simulink model "fs9_sim_sdr_v0"  (R2022b)
settings: Solver=ode4  StartTime=0.0  StopTime=dm.duration  FixedStep=dm.dt  RelTol=1e-3
PreLoadFcn:
  | addpath('./Common');
  | addpath('./design_tuning');
  | addpath('./sim_config');
  | addpath('./sim_analysis');
  | addpath('./fsw_init');
  | addpath('./mdls');
  | rads2rpm    = 60/(2*pi);  %rad/s to rpm
  | deg2rad     = pi/180;
  | set_mdl_variant;
InitFcn:
  | %b5g_init_param_sdr_v1;
model workspace (MAT data in the model file):
  RWModelType = 0
undefined symbols (not defined in the file or in its folder): dm, Eclipse, fsw, MagSc, mdl, PVeci, Qi2b, RateSc, SunSc
libraries: simulink x3, vrlib x2, aerolibtransform2 x1
(part 2 of 2)

== stateflow chart fs9_sim_sdr_v0/Manager & Control/AOCS_FSW ==
  state AOCS_MGR
    tcur = elapsed(sec);
    exec_ttc;
    state NM
      state NM_MGR [parallel]
        en,du:
        sun_direction_proc;
        eclipse_proc;
        settings: executionOrder=1
        state OFF
        state SUP
          en,du:
          GUIDANCE.set_sun_dir(sun_dir);
          sup_trans_count;
        state GAP
          gap_trans_count;
        state MAN
        state FIP
        (default) -> AOCS_MGR.NM.NM_MGR.OFF
        AOCS_MGR.NM.NM_MGR.OFF -> AOCS_MGR.NM.NM_MGR.GAP [order 2] : [C2]{A5}
        AOCS_MGR.NM.NM_MGR.OFF -> AOCS_MGR.NM.NM_MGR.SUP [order 1] : [C1]{A4}
        AOCS_MGR.NM.NM_MGR.GAP -> AOCS_MGR.NM.NM_MGR.SUP [order 1] : [C1]{A4}
        AOCS_MGR.NM.NM_MGR.SUP -> AOCS_MGR.NM.NM_MGR.GAP [order 1] : [C2]{A5}
        AOCS_MGR.NM.NM_MGR.FIP -> AOCS_MGR.NM.NM_MGR.GAP [order 3] : GO_HOME[C2]{A5}
        AOCS_MGR.NM.NM_MGR.GAP -> AOCS_MGR.NM.NM_MGR.MAN [order 2] : SWITCH_MAN[C3]{A2}
        AOCS_MGR.NM.NM_MGR.SUP -> AOCS_MGR.NM.NM_MGR.MAN [order 2] : SWITCH_MAN[C3]{A2;}
        AOCS_MGR.NM.NM_MGR.FIP -> AOCS_MGR.NM.NM_MGR.SUP [order 2] : GO_HOME[C1]{A4}
        AOCS_MGR.NM.NM_MGR.FIP -> AOCS_MGR.NM.NM_MGR.MAN [order 1] : SWITCH_MAN[C3]{A2}
        AOCS_MGR.NM.NM_MGR.MAN -> AOCS_MGR.NM.NM_MGR.FIP : [C4]{A3}
      state GUIDANCE [parallel]
        settings: executionOrder=2
        state OFF
        state GAP
          en,du:
          gap_proc;
        state SUP
          en,du:
          gap_proc;
          %sup_proc;
        state MAN
          en,du:
          man_proc;
        state FIP
          fip_proc;
        (default) -> AOCS_MGR.NM.GUIDANCE.OFF
        AOCS_MGR.NM.GUIDANCE.OFF -> AOCS_MGR.NM.GUIDANCE.SUP [order 2] : SWITCH_SUP{A1}
        AOCS_MGR.NM.GUIDANCE.OFF -> AOCS_MGR.NM.GUIDANCE.GAP [order 1] : SWITCH_GAP{A2}
        AOCS_MGR.NM.GUIDANCE.GAP -> AOCS_MGR.NM.GUIDANCE.SUP [order 1] : SWITCH_SUP{A1}
        AOCS_MGR.NM.GUIDANCE.SUP -> AOCS_MGR.NM.GUIDANCE.GAP [order 1] : SWITCH_GAP{A2}
        AOCS_MGR.NM.GUIDANCE.FIP -> AOCS_MGR.NM.GUIDANCE.GAP [order 2] : SWITCH_GAP{A2}
        AOCS_MGR.NM.GUIDANCE.GAP -> AOCS_MGR.NM.GUIDANCE.MAN [order 2] : SWITCH_MAN{A3}
        AOCS_MGR.NM.GUIDANCE.FIP -> AOCS_MGR.NM.GUIDANCE.SUP [order 3] : SWITCH_SUP{A1}
        AOCS_MGR.NM.GUIDANCE.SUP -> AOCS_MGR.NM.GUIDANCE.MAN [order 2] : SWITCH_MAN{A3}
        AOCS_MGR.NM.GUIDANCE.FIP -> AOCS_MGR.NM.GUIDANCE.MAN [order 1] : SWITCH_MAN{A3}
        AOCS_MGR.NM.GUIDANCE.MAN -> AOCS_MGR.NM.GUIDANCE.FIP : SWITCH_FIP{A4}
      state NM_CONTROL [parallel]
        settings: executionOrder=3
        state WHEEL_ONLY
          en, du:
          pre_proc;
          wheel_control_proc;
          wheel_off_loading_proc;
        state OFF
        (default) -> AOCS_MGR.NM.NM_CONTROL.OFF
        AOCS_MGR.NM.NM_CONTROL.OFF -> WHEEL_ONLY
    state ASH_MGR
      state ASH [parallel]
        du:
        ASH_MGR_RTC;
        settings: executionOrder=1
        state IDLE
        state STABILIZE
          entry, during:
          stabilize_processing;
        state SLO
          entry,during:
          sun_lock_processing;
          wheel_off_loading_proc
          if ~sun_presence
          count_day_night =  count_day_night+1;
          else
          count_day_night = 0;
          end
        state STRA
          during:
          if sun_presence
          count_day_night =  count_day_night+1;
          else
          count_day_night = 0;
          end
        (default) -> IDLE
        IDLE -> STABILIZE : [C1]{A1}
        STABILIZE -> STRA : [C2]{A2}
        STRA -> SLO : [C3]{A3}
        SLO -> STRA : [C4]{A4}
      state ASH_CTRL [parallel]
        du:
        ASH_CTRL_RTC
        settings: executionOrder=2
        state OFF
        state MTQ_ONLY
          entry, during:
          RW_FUN   = ...
          rw_momentum_control(SENSOR_IN.Hrw);
          MTQ_FUN = ...
          magnetic_control(SENSOR_IN.MAG_FUNC)
          exit:
          MTQ_FUN = zeros(3,1);
        state MTQ_AND_RW
          entry,during:
          RW_FUN = ...
          sunsensor_control(SENSOR_IN.SS_FUNC,...
          SENSOR_IN.rate_est );
        (default) -> AOCS_MGR.ASH_MGR.ASH_CTRL.OFF
        AOCS_MGR.ASH_MGR.ASH_CTRL.OFF -> MTQ_ONLY : SCHEDULE_OBJECT
        MTQ_ONLY -> MTQ_AND_RW : SELECT_MTQ_AND_RW
        MTQ_AND_RW -> MTQ_ONLY : SELECT_MTQ_ONLY
      state rw_cmd = rw_momentum_control(HrwEst) [function]
      state stop_sim [function]
      state mtq_cmd = magnetic_control(MAG_FUNC) [function]
      state rw_cmd = sunsensor_control(ss_tm,iru_tm) [function]
    (default) -> (junction 132)
    (junction 132) -> (junction 135) [order 2]
    (junction 132) -> NM [order 1] : [AOCS_MODE==1]
    (junction 135) -> ASH_MGR
  data: C function_output; C function_output; C function_output; C function_output; sat_in_eclipse local boolean size=1 =false; object_state local Enum: NMMODE size=1 =NMMODE.OFF; sun_dir local double size=3 =[1 0 0]'; gap_sup_counter local double size=1 =0; steady_count local double size=1 =0; sup_gap_counter local double size=1 =0; dt function_output; C function_output; C function_output; Q function_output; W function_output; A function_output; sv function_input; qin function_input; dt function_input; object_state local Enum: GUIDMODE size=1 =GUIDMODE.OFF; sun_dir local double size=3 =[1 0 0]';; Qin2cons local double size=4 =[1 0 0 0]';; Wcons local double size=3 =[0 0 0]'; Acons local double size=3 =[0 0 0]'; Qlvlh2cons_end local double size=4 =[1 0 0 0]'; dt_man local double size=1 =0; man_feasibility_flag local boolean size=1 =false; theta_rot local double size=1 =0; Amax local double size=1 =0; end_of_man_flag local boolean size=1 =false; t_curr local double size=1 =0; Acurr local double size=1 =0; Wcurr local double size=1 =0; theta_curr local size=1 =0; Qlvlh2cons_fip local double size=4 =[1 0 0 0]'; Qin2sat_init local double size=4 =[1 0 0 0]'; T_VHF local double size=1 =fsw.dt; axis_rot local double size=3 =[1 0 0]'; T1 local double size=1 =0; T2 local double size=1 =0; Wrot local double size=1 =0; da function_output; dr function_output; Hrw local double size=3 =[0 0 0]'; Qerr local double size=4 =[1 0 0 0]'; d_theta local double size=3 =[0 0 0]'; d_omega local double size=3 =[0 0 0]'; Acons local double size=3 =[0 0 0]'; Wcons local double size=3 =[0 0 0]'; Qin2cons local double size=4 =[1 0 0 0]'; West local double size=3 =[0 0 0]'; rate_bias local double size=3 =[0 0 0]'; B0 local double size=3 =[0 0 0]'; maxB local double size=1; C function_output boolean size=1; HrwEst function_input double size=3; rw_cmd function_output; C function_output; MAG_FUNC function_input double size=9; mtq_cmd function_output; C function_output; ss_tm function_input double size=4; iru_tm function_input double size=3; rw_cmd function_output; C function_output; object_state local Enum: ASHMODE size=1; tcur local double size=1 =0; fsw parameter; count_stab local double size=1; count_day_night local double size=1 =0; SENSOR_IN input Bus: SENSORS; stabilized local boolean size=1; stabilize_duration local double; sun_mislocked_duration local double size=1 =0; sun_locked_duration local double size=1 =0; sun_presence local boolean size=1 =false; RW_FUN output double size=3 =zeros(3,1); MTQ_FUN output double size=3 =zeros(3,1); AOCS_MODE local double size=1 =fsw.aocs_mode; udot_norm local double size=1 =0
  data udot_norm settings: description=log data
  events: SWITCH_MAN local FUNCTION_CALL_EVENT; GO_HOME local FUNCTION_CALL_EVENT; SWITCH_SUP local FUNCTION_CALL_EVENT; SWITCH_GAP local FUNCTION_CALL_EVENT; SWITCH_MAN local FUNCTION_CALL_EVENT; SWITCH_FIP local FUNCTION_CALL_EVENT; SELECT_MTQ_AND_RW local FUNCTION_CALL_EVENT; SELECT_MTQ_ONLY local FUNCTION_CALL_EVENT; SCHEDULE_OBJECT local FUNCTION_CALL_EVENT
  function C = C1:
    | function C = C1
    | C = sat_in_eclipse== false;
  function C = C2:
    | function C = C2
    | C = sat_in_eclipse== true;
  function C = C3:
    | function C = C3
    | C = GUIDANCE.get_man_feasibility_flag;
  function C = C4:
    | function C = C4
    | C = GUIDANCE.get_end_of_man_flag;
  function A2:
    | function A2
    | send(GUIDANCE.SWITCH_MAN, GUIDANCE);
    | object_state = NMMODE.MAN;
  function A3:
    | function A3
    | 
    | send(GUIDANCE.SWITCH_FIP, GUIDANCE);
    | object_state = NMMODE.FIP;
  function A4:
    | function A4
    | send(GUIDANCE.SWITCH_SUP, GUIDANCE);
    | object_state = NMMODE.SUP;
    | sup_gap_counter = 0;
  function A5:
    | function A5
    | 
    | send(GUIDANCE.SWITCH_GAP, GUIDANCE);
    | object_state = NMMODE.GAP;
    | gap_sup_counter = 0;
  function eclipse_proc:
    | function eclipse_proc
    | 
    | p_sat_eci = SENSOR_IN.pvt_eci_nav(1:3);
    | 
    | if dot(p_sat_eci, sun_dir) > fsw.nm_mgr.eclipse_param
    |     sat_in_eclipse = false;
    | else
    |     sat_in_eclipse = true;
    | end
  function sun_direction_proc:
    | function sun_direction_proc
    | jD = SENSOR_IN.pvt_eci_nav(7);
    | T = JDCentury(jD);
    | lamda_mean     = rem(280.460+36000.771*T,360);
    | mean_anomaly   = rem(357.5291092+35999.05034*T,360);
    | lamda_ecliptic = lamda_mean+ 1.914666471*sind(mean_anomaly)...
    |                  + 0.019994643*sind(2*mean_anomaly);
    | % Obliquity of ecliptic
    | epsilon = 23.439291 -0.0130042*T;
    | sun_dir  = [cosd(lamda_ecliptic);...
    |            cosd(epsilon)*sind(lamda_ecliptic);...
    |            sind(epsilon)*sind(lamda_ecliptic)];
  function sup_trans_count:
    | function sup_trans_count
    | [ang_err, ~] = NM_CONTROL.get_control_error;
    | ang_max = max(abs(ang_err));
    | if ang_max >= fsw.nm_mgr.ang_thd
    |     gap_sup_counter = gap_sup_counter + fsw.dt;
    |     if steady_count ~= 0
    |         steady_count = 0;
    |     end
    | else
    |      if steady_count <=  fsw.nm_mgr.Tsteady
    |          gap_sup_counter = gap_sup_counter + fsw.dt;
    |          steady_count    = steady_count + fsw.dt;
    |      else
    |          gap_sup_counter = 0;
    |      end
    | end
  function gap_trans_count:
    | function gap_trans_count
    | [ang_err, ~] = NM_CONTROL.get_control_error;
    | ang_max = max(abs(ang_err));
    | if ang_max >= fsw.nm_mgr.ang_thd
    |     sup_gap_counter = sup_gap_counter + fsw.dt;
    |     if steady_count ~= 0
    |         steady_count = 0;
    |     end
    | else
    |      if steady_count <=  fsw.nm_mgr.Tsteady
    |          sup_gap_counter = sup_gap_counter + fsw.dt;
    |          steady_count    = steady_count + fsw.dt;
    |      else
    |          sup_gap_counter = 0;
    |      end
    | end
  function dt = make_fesability:
    | function dt = make_fesability
    |  
    | Qi2bInit   = SENSOR_IN.qi2b_est;
    | Qi2l       = SENSOR_IN.nav_out(4:7);
    | Isat       = fsw.EstIb;
    | G          = fsw.rw.func.G;
    | DHalloc    = fsw.guid.WHEEL_MOM_ALLOC;
    | TrwMax     = fsw.guid.WHEEL_MAX_TORQUE;
    | Wthd       = fsw.guid.MAN_ANG_RATE_SAT;
    | 
    | Qi2consEnd = QMul(Qi2l, Qlvlh2cons_end);
    | 
    | Qman       = QMul(QInv(Qi2bInit), Qi2consEnd);
    | Qman       = QNormal(Qman);
    | 
    | if Qman(1) <0
    |     Qman = -Qman;
    | end
    | theta_rot = 2 * acos(Qman(1));
    | 
    | if theta_rot < fsw.guid.EPSILON_MAN
    |     theta_rot = 0;
    |     axis_rot  =[1 0 0]';
    | else
    |     axis_rot = Qman(2:4)/sqrt(1-Qman(1)^2);
    | end
    | 
    | Acc         = abs(G*Isat*axis_rot);
    | dh_over_a   = [inf inf inf inf]';
    | tmax_over_a = [inf inf inf inf]';
    | for i=1:4
    |     if Acc(i)~=0
    |         dh_over_a(i)  = DHalloc(i)/Acc(i);
    |         tmax_over_a(i)= TrwMax(i)/Acc(i);
    |     end
    | end
    | Wmax = min([dh_over_a' Wthd]);
    | Amax = min(tmax_over_a);
    | 
    | %% step 4 
    | if theta_rot <= Wmax^2/Amax
    |     dt = sqrt(4*theta_rot/Amax);
    | else
    |     dt = (theta_rot/Wmax+Wmax/Amax); %(theta_rot+Wmax^2/Amax)/Wmax
    | end
    | dt    = ceil(dt);
    | 
    | end
  function C = get_end_of_man_flag:
    | function C = get_end_of_man_flag
    |  
    | C = end_of_man_flag;
  function C = get_man_feasibility_flag:
    | function C = get_man_feasibility_flag
    | if dt_man == 0
    |    fprintf('dt_man: ');
    |    dt_man  = make_fesability;
    |    fprintf('%.1f, ',dt_man);
    |    check_man_feasibility_proc;
    |    while (~man_feasibility_flag)
    |        dt_man = dt_man+1;
    |        check_man_feasibility_proc;
    |        fprintf('%.1f, ',dt_man);
    |    end
    |    fprintf('\n');
    | end
    | check_man_feasibility_proc;
    | C = man_feasibility_flag;
  function [Q, W, A] = get_guid_data:
    | function [Q, W, A]=get_guid_data
    | A = Acons;    
    | Q = Qin2cons ;
    | W = Wcons ;   
    | end
  function set_sun_dir(sv):
    | function set_sun_dir(sv)
    | sun_dir = sv;
  function set_man_profile(qin, dt):
    | function set_man_profile(qin, dt)
    | Qlvlh2cons_end    = qin;
    | dt_man            = dt;
    | end
  function check_man_feasibility_proc:
    | function check_man_feasibility_proc
    | 
    | Isat    = fsw.EstIb;
    | G       = fsw.rw.func.G;
    | DHalloc = fsw.guid.WHEEL_MOM_ALLOC;
    | TrwMax  = fsw.guid.WHEEL_MAX_TORQUE;
    | Wthd    = fsw.guid.MAN_ANG_RATE_SAT;
    | Omega   = SENSOR_IN.nav_out(1:3);
    | 
    | Qlvlh_init2end = [cos(Omega(2)*dt_man/2); 0;...
    |                   sin(Omega(2)*dt_man/2); 0];
    | 
    | Qin2lvlh       = SENSOR_IN.nav_out(4:7);
    | 
    | Qin2cons_end   = QMul(QMul(Qin2lvlh, Qlvlh_init2end), Qlvlh2cons_end);
    | Qin2sat_init   = SENSOR_IN.qi2b_est;
    | Qman           = QMul(QInv(Qin2sat_init), Qin2cons_end);
    | Qman           = QNormal(Qman);
    | 
    | if Qman(1) <0
    |         Qman = -Qman;
    | end
    | 
    | if Qman(1) > 1 
    |     man_feasibility_flag = false;
    |     return;
    | end
    | 
    | theta_rot = 2 * acos(Qman(1));
    | 
    | if theta_rot < fsw.guid.EPSILON_MAN
    |     theta_rot = 0;
    |     axis_rot  =[1 0 0]';
    | else
    |     axis_rot = Qman(2:4)/sqrt(1-Qman(1)^2);
    | end
    | 
    | Acc         = abs(G*Isat*axis_rot);
    | dh_over_a   = [inf inf inf inf]';
    | tmax_over_a = [inf inf inf inf]';
    | for i=1:4
    |     if Acc(i)~=0
    |         dh_over_a(i)  = DHalloc(i)/Acc(i);
    |         tmax_over_a(i)= TrwMax(i)/Acc(i);
    |     end
    | end
    | Wmax = min([dh_over_a' Wthd]);
    | Amax = min(tmax_over_a);
    | 
    | if dt_man < fsw.dt || Amax == 0
    |     man_feasibility_flag = false;
    |     
    | elseif dt_man <= 2*Wmax/Amax && theta_rot<=Amax*dt_man^2/4
    |     man_feasibility_flag = true;
    |     
    | elseif dt_man >= 2*Wmax/Amax && theta_rot<=Wmax*dt_man-Wmax^2/Amax
    |     man_feasibility_flag = true;
    |     
    | else
    |     man_feasibility_flag = false;
    | end
    | 
    | % if(~man_feasibility_flag)
    | %     disp('MAN Failed');
    | % end
  function man_proc:
    | function man_proc
    | 
    | if t_curr >= dt_man
    |     Acurr = 0;
    |     Wcurr = 0;
    |     theta_curr = theta_rot;
    |     end_of_man_flag = true;
    | elseif t_curr >= T2 && t_curr < dt_man
    |     Acurr = -Amax;
    |     Wcurr = Amax*(dt_man - t_curr);
    |     theta_curr = theta_rot - 0.5*Amax * (dt_man - t_curr)^2;
    |  elseif t_curr >= T1 && t_curr < T2
    |     Acurr = 0;
    |     Wcurr = Wrot;
    |     theta_curr = theta_rot/2 + Wrot * (t_curr - dt_man/2);
    | elseif t_curr < T1
    |     Acurr = Amax;
    |     Wcurr = Amax * t_curr;
    |     theta_curr = 0.5*Amax * t_curr^2;
    | end    
    | Qsat2cons_curr = [cos(theta_curr/2);sin(theta_curr/2).*axis_rot];
    | Qin2cons = QMul(Qin2sat_init,Qsat2cons_curr);
    | Wcons = Wcurr.*axis_rot;
    | Acons = Acurr.*axis_rot;
    | t_curr = t_curr + T_VHF;
    |     
    | end
  function fip_proc:
    | function fip_proc
    | 
    | Qin2lvlh = SENSOR_IN.nav_out(4:7);
    | Qin2cons = QMul(Qin2lvlh, Qlvlh2cons_fip);
    | 
    | Worb = SENSOR_IN.nav_out(1:3);
    | 
    | q_temp = QMul(QMul(QInv(Qlvlh2cons_fip),[0;Worb]), Qlvlh2cons_fip);
    | Wcons  = q_temp(2:4);
    |     
    | end
  function gap_proc:
    | function gap_proc
    | Acons    = zeros(3,1);
    | Qin2cons = SENSOR_IN.nav_out(4:7);
    | Wcons    = SENSOR_IN.nav_out(1:3);
    | end
  function sup_proc:
    | function sup_proc()
    | 
    | if fsw.guid.SUP_SLEW_MODE
    |     Qin2cons = sun_sync_sup_slew;
    | else
    |     Qin2cons = dir_sup_slew;
    | end
    | Wcons = zeros(3,1);
    | Acons = zeros(3,1);
    | end
    | 
    | function QuatSup = sun_sync_sup_slew
    |     Qi2l = SENSOR_IN.nav_out(4:7);
    |     SunEci = sun_dir;
    |     Qorb = QMul(Qi2l,QMul([0 0 1 0]',QInv(Qi2l)));
    |     Norb = Qorb(2:4);
    |     Ux   = cross(Norb,SunEci);
    |     Ux   = Ux/norm(Ux);
    |     if(Ux(3)>0)
    |         Ux = -Ux;
    |     end
    |     Uz   = -SunEci;
    |     Uy   = cross(Uz,Ux);
    |     QuatSup = M2Q([Ux Uy Uz]);
    | end
    | 
    | 
    | function QuatSup = dir_sup_slew
    |     Qin2sat = SENSOR_IN.qi2b_est;
    |     SunEci  = sun_dir;
    |     Qsb = QMul(QInv(Qin2sat),QMul([0;SunEci],Qin2sat));
    |     SunBody = Qsb(2:4);
    |     prj = dot([0 0 -1]', SunBody);
    |     if prj >1 || prj< -1
    |         prj = 1;
    |     end
    |     dlt_ang = acos(prj);
    |     rotAxis = cross([0 0 -1]', SunBody);
    |     rotAxis = rotAxis/norm(rotAxis);
    |     Qb2c = [cos(dlt_ang/2); rotAxis*sin(dlt_ang/2)];
    |     QuatSup = QMul(Qin2sat,Qb2c);
    | end
  function A1:
    | function A1
    | 
    | object_state = GUIDMODE.SUP;
  function A2:
    | function A2
    | 
    | object_state = GUIDMODE.SUP;
  function A3:
    | function A3
    | 
    | object_state = GUIDMODE.MAN;
    | 
    | %% initialization of man proc
    | alpha  = 1 - sqrt(1 - 4*theta_rot/(Amax*dt_man^2));
    | T1     = alpha*dt_man/2;
    | T2     = dt_man-T1;
    | Wrot   = alpha * Amax *dt_man/2;
    | T1     = alpha*dt_man/2;
    | T2     = dt_man-T1;
    | Wrot   = alpha * Amax *dt_man/2;
    | end_of_man_flag = false;
    | t_curr = 0;
    | Qlvlh2cons_fip = Qlvlh2cons_end;
  function A4:
    | function A4
    | 
    | object_state = GUIDMODE.FIP;
    | Acons = zeros(3,1);
  function pre_proc:
    | function pre_proc()
    | Qin2sat = SENSOR_IN.qi2b_est;
    | West    = SENSOR_IN.rate_est;
    | Hrw     = SENSOR_IN.Hrw;
    | 
    | [Qin2cons, Wcons, Acons] = GUIDANCE.get_guid_data;
    | deltaQ = QMul(QInv(Qin2cons),Qin2sat);
    | if deltaQ(1)<0
    |         deltaQ = deltaQ *-1;
    | end
    | 
    | d_theta = 2.0*deltaQ(2:4);
    | d_omega = West-Wcons;
    | Qerr = QNormal(deltaQ);
    | 
    | end
  function wheel_off_loading_proc:
    | function wheel_off_loading_proc
    | Isat = fsw.EstIb;
    | B = SENSOR_IN.MAG_FUNC(7:9);
    | Htot = Isat*West + Hrw;
    | % delta_h = (Hrw + fsw.Ib*RateEst) - fsw.rw.func.h_ref;
    | delta_h = Htot - fsw.ctrl.h_ref;
    | m = cross(B,delta_h)*(-fsw.ctrl.off_load_ctrl_gain/norm(B)^2);
    | m_max = max(abs(m));
    | if m_max  > fsw.mtq.func.max_dipole
    |     m = m*(fsw.mtq.func.max_dipole/m_max) ;
    | end
    |     
    | MTQ_FUN = m;
    | end
  function wheel_control_proc:
    | function wheel_control_proc
    | Kv = fsw.ctrl.KD;
    | Ke = fsw.ctrl.KP;
    | Isat = fsw.EstIb;
    | % if Qerr(1)==1
    | %     disp('divided by zeros');
    | % end
    | if dot(Qerr(2:4),Qerr(2:4)) > 0.25 * fsw.ctrl.thet_thd^2
    |    if Qerr(1)==1
    |        B0 = zeros(3,1);
    |    else
    |        Bdir = Qerr(2:4)/norm(Qerr(2:4));
    |        B0 = -fsw.ctrl.RateBiasMaxNorm*Bdir;
    | %        B0 = -(fsw.ctrl.RateBiasMaxNorm/sqrt(1-Qerr(1)^2)).*Qerr(2:4);
    | %        disp(Qerr(2:4));
    |    end
    |    maxB = max([1;abs(B0)./fsw.ctrl.RateBiasMax]);
    |    rate_bias = B0/maxB;  
    |    Trw = Isat*(Kv.*(d_omega - rate_bias));
    |    Tol = zeros(3,1);
    | else
    |    rate_bias = zeros(3,1);
    |    Trw = Isat*(Ke.*d_theta + Kv.*d_omega); 
    |    Tol  = Isat*Acons + cross(Wcons, Isat*Wcons + Hrw);
    | end
    | 
    | RW_FUN = Trw - Tol;
    | 
    | end
  function [da ,dr] = get_control_error:
    | function [da ,dr] = get_control_error
    | da = d_theta;
    | dr = d_omega;
  function stabilize_processing:
    | function stabilize_processing
    | 
    | udot = SENSOR_IN.MAG_FUNC(1:3);
    | udot_norm = norm(udot);
    | 
    | if  udot_norm < fsw.ash_mgr.epsilon
    |     count_stab = count_stab+1;
    | else
    |     count_stab = 0;
    | end
    | if count_stab > fsw.ash_mgr.Tstab
    |     stabilized = true;
    |     if fsw.ash_mgr.stop_once_stab
    |         stop_sim;
    |     end
    | end
  function A1:
    | function A1
    | 
    | count_stab = 0;
    | stabilized = false;
    | stabilize_duration = 0;
    | send(ASH_CTRL.SCHEDULE_OBJECT, ASH_CTRL.OFF);
    | 
    | 
    | ASH_MGR.object_state = ASHMODE.STAB;
  function C = C1:
    | function C = C1
    | % Check that all necessary equipments for the STABILIZE submode are ON
    | C = true;
  function ASH_CTRL_RTC:
    | function ASH_CTRL_RTC
    | 
    | if ~in(ASH_CTRL.MTQ_AND_RW)
    |     sunsensor_control(SENSOR_IN.SS_FUNC, SENSOR_IN.rate_est );
    | end
  function sun_lock_processing:
    | function sun_lock_processing
    | 
    | sun_locked_duration = sun_locked_duration + 1;
  function C = C2:
    | function C = C2
    | C = stabilized;%stablized;
  function A2:
    | function A2
    | ASH_MGR.object_state = ASHMODE.STRA;
    | count_day_night = 0;
  function wheel_off_loading_proc:
    | function wheel_off_loading_proc
    | 
    | West    = SENSOR_IN.rate_est;
    | Hrw     = SENSOR_IN.Hrw;
    | Isat = fsw.EstIb;
    | B = SENSOR_IN.MAG_FUNC(7:9);
    | Htot = Isat*West + Hrw;
    | % delta_h = (Hrw + fsw.Ib*RateEst) - fsw.rw.func.h_ref;
    | delta_h = Htot - fsw.rw.func.h_ref;
    | m = cross(B,delta_h)*(-fsw.rw.func.off_load_ctrl_gain/norm(B)^2);
    | 
    | 
    | m_max = max(abs(m));
    | if m_max  > fsw.mtq.func.max_dipole
    |     m = m*(fsw.mtq.func.max_dipole/m_max) ;
    | end
    |         
    | MTQ_FUN = m/5;%@@
    | end
  function ASH_MGR_RTC:
    | function ASH_MGR_RTC
    | 
    | sun_presence = ...
    |     boolean(SENSOR_IN.SS_FUNC(4));
    | ASH_MGR.object_state = ...
    |     ASH_MGR.object_state;
    | 
    | % count_stab = count_stab;
  function C = C3:
    | function C = C3
    | C = count_day_night >= fsw.ash_mgr.Tconf;
  function A3:
    | function A3
    | 
    | % send(ASH_CTRL.SELECT_MTQ_AND_RW, ASH_CTRL.MTQ_ONLY);
    | ASH_MGR.object_state = ASHMODE.SLO;
    | count_day_night = 0;
    | 
    | sun_locked_duration = 0;
    | sun_mislocked_duration = 0;
  function C = C4:
    | function C = C4
    | C = count_day_night >= fsw.ash_mgr.Tconf;
  function A4:
    | function A4
    | 
    | % send(ASH_CTRL.SELECT_MTQ_ONLY, ASH_CTRL.MTQ_AND_RW);
    | % send(ASH_CTRL.SELECT_MTQ_AND_RW, ASH_CTRL.MTQ_ONLY);
    | % 
    | % send(ASH_CTRL.SELECT_MTQ_ONLY, ASH_CTRL.MTQ_AND_RW);
    | ASH_MGR.object_state = ASHMODE.STRA;
    | count_day_night = 0;
    | count_stab = 0;
    | stabilized = false;
  function exec_ttc:
    | function exec_ttc
    | if isempty(fsw.ttc)
    |     return;
    | end
    | ttc = fsw.ttc;
    | num = size(ttc,2);
    | % disp(elapsed('sec'));
    | for i=1:num
    |     if (ttc(i).exec_time == tcur)
    |         switch ttc(i).type
    |             case TTC.GO_HOME
    |                 fprintf('%.2f : GO HOME\n',tcur);
    |                 send(NM.NM_MGR.GO_HOME, NM.NM_MGR);
    |             case TTC.SWITCH_MAN
    |                 NM.GUIDANCE.set_man_profile(ttc(i).q_lvlh2cons, ttc(i).dt);
    |                 ra = asind(ttc(i).q_lvlh2cons(2:4))*2;
    |                 fprintf('%.2f : MAN (%.1f, %.1f, %.1f) in %.1f sec\n',...
    |                        tcur,ra(1), ra(2), ra(3), ttc(i).dt );
    |                 send(NM.NM_MGR.SWITCH_MAN, NM.NM_MGR);
    |         end
    |     end
    |  
    | end

== matlab function fs9_sim_sdr_v0/Space Environment Models/Eclipse Condition ==
  data: SunEci input; EclipFlag output; PvEci input
function EclipFlag  = Eclipse(SunEci, PvEci)
Dp = -PvEci(1:3)*1e-3;  % earth vector in Km
Rp = 6378.137;          % earth radius in km
Rs = 6.9599e5;          % solar photosphere radius in km
S  = 1.49597870e8;      % astronomical unit in km
C  = 1.385e6;           % size of earth shadow cone
Ds = (S.*SunEci + Dp);  % vector from S/C to the Sun

DsNorm = norm(Ds);
DpNorm = norm(Dp);
rho_s  = asind(Rs/DsNorm);
rho_p  = asind(Rp/DpNorm);
theta  = acosd(dot(Ds, Dp) / (DsNorm * DpNorm));
if ( theta < (rho_p - rho_s) && DsNorm > S && (S + C) > DsNorm)
    EclipFlag = 1;
else
	EclipFlag = 0;
end

== matlab function fs9_sim_sdr_v0/Space Environment Models/Sun Model ==
  data: jD input; SunEci output
function SunEci = SunModel(jD)
T = JDCentury(jD);
lamda_mean     = rem(280.460+36000.771*T,360);
mean_anomaly   = rem(357.5291092+35999.05034*T,360);
lamda_ecliptic = lamda_mean+ 1.914666471*sind(mean_anomaly)...
                 + 0.019994643*sind(2*mean_anomaly);
% Obliquity of ecliptic
epsilon = 23.439291 -0.0130042*T;
SunEci  = [cosd(lamda_ecliptic);...
           cosd(epsilon)*sind(lamda_ecliptic);...
           sind(epsilon)*sind(lamda_ecliptic)];

== matlab function fs9_sim_sdr_v0/Manager & Control/AOCS_FSW/AOCS_MGR.ASH_MGR.magnetic_control/Bdot Control ==
  settings: updateMethod=DISCRETE
  data: MAG_FUNC input; Mc output; fsw parameter
%% Bdot Control Rev
function Mc  = Bdot(MAG_FUNC, fsw)

sdot  =  MAG_FUNC(4:6);
Mc    = -fsw.bdot_gain.*sdot;

end

== matlab function fs9_sim_sdr_v0/NAV & IAE/NAVIGATION ==
  data: pvt_eci input; nav_out output; pvt_eci_nav output; fsw parameter
function [nav_out, pvt_eci_nav]  = Navgation(pvt_eci, fsw)

p_nav = pvt_eci(1:3) + fsw.nav.p_noise*randn(3,1)*fsw.nav.noise_enable;
v_nav = pvt_eci(4:6) + fsw.nav.v_noise*randn(3,1)*fsw.nav.noise_enable;

omega_orbit = OrbitPusaltion(pvt_eci);
Qi2l        = PVi2Qi2l(pvt_eci);
nav_out     = [omega_orbit; Qi2l];
pvt_eci_nav  = [p_nav ;v_nav;pvt_eci(7)];

== matlab function fs9_sim_sdr_v0/Manager & Control/AOCS_FSW/AOCS_MGR.ASH_MGR.sunsensor_control/SunAngErr ==
  data: deltaAngle_c2b output; snr_fun input
function deltaAngle_c2b = RPLD_CTRL_PROC(snr_fun)

if ~snr_fun(4) 
    deltaAngle_c2b = [0;0;0];
    return;
end

vec_sun_b = snr_fun(1:3);
mag = norm(vec_sun_b);
if mag~=0
    vec_sun_b = vec_sun_b/mag;
end

%% DCM to Euler Angle Method
zb = (-1)*vec_sun_b';
yb = [0 vec_sun_b(3) -vec_sun_b(2)];
xb = cross(yb,zb);
R_B2C = [xb;yb;zb];

theta_c2b = -asin(R_B2C(3, 1));
phi_c2b = atan(R_B2C(3, 2) / R_B2C(3, 3));
% psi_c2b = atan2(R_B2C(2, 1), R_B2C(1, 1)); //3.14
psi_c2b = atan(R_B2C(2, 1) / R_B2C(1, 1));

%% deltaAngle_c2b = deltaAngle_b/c = -deltaAngle_c/b = -deltaAngle_b2c
deltaAngle_c2b = [phi_c2b; theta_c2b; psi_c2b];

== matlab function fs9_sim_sdr_v0/NAV & IAE/Inertial Attitude Estimation ==
  settings: updateMethod=DISCRETE
  data: Qi2b_true input; Q2ib output; RateSc_true input; RateSc output; fsw parameter
function [Q2ib, RateSc]= IAE(Qi2b_true, RateSc_true, fsw)

if fsw.iae.noise_enable
    dltQ   = (fsw.iae.att_noise.*randn(3,1)/2)*fsw.iae.noise_enable;
    qNoise = [sqrt(1-dltQ'*dltQ);dltQ];
    Q2ib   = QUnit(QMul(Qi2b_true, qNoise));
else
    Q2ib   = Qi2b_true;
end
RateSc = RateSc_true + fsw.iae.rate_noise*randn(3,1)*fsw.iae.noise_enable;

== matlab function fs9_sim_sdr_v0/MTQ_FUN/MATLAB Function ==
  data: Mc input; duty output double; fsw parameter
function duty = fcn(Mc, fsw)
max_dipole = fsw.mtq.func.max_dipole;
mtq_period = fsw.mtq.cycle;
Mm = Mc;
mx = max(abs(Mc));
if mx>max_dipole
    Mm = Mm*(max_dipole/mx);
end

duty = Mm*(mtq_period-1)/(max_dipole*mtq_period);

== matlab function fs9_sim_sdr_v0/Sensor Modeling/ZARM FGM-A-75 ==
  settings: updateMethod=DISCRETE
  data: MagScTrue input; MagScNoise output; dm parameter
function MagScNoise = fcn(MagScTrue, dm)

if dm.mag_mdl.enable_noise

    mag_norm_ture = norm(MagScTrue);
    if abs(mag_norm_ture-eps) < 10*eps
        MagScNoise = MagScTrue;
        return;
    end
    mag_dir_true  = MagScTrue/mag_norm_ture;
    
    
    
    rdn_dir = [randn(2,1);0];        % only for x and y axis
    rdn_dir = rdn_dir/norm(rdn_dir);
    thet_dist = dm.mag_mdl.ang_err*randn(1,1)/2; %half noise
    
    q_dist = [cos(thet_dist); rdn_dir*sin(thet_dist)];
    
    mag_dir_dist = QMul([0;mag_dir_true],q_dist);
    mag_norm_dist = mag_norm_ture*(1 + dm.mag_mdl.norm_err*randn(1,1));
    
    mag_dist = mag_dir_dist(2:4)*mag_norm_dist;
    
    MagScNoise = mag_dist + dm.mag_mdl.noise * randn(3,1)...
                          + dm.mag_mdl.linerity_err * randn(3,1)...
                          + dm.mag_mdl.offset_err * randn(3,1);

else
    MagScNoise = MagScTrue;
end

== matlab function fs9_sim_sdr_v0/Spacecraft/Spacecraft Dynamics/Disturbance Models/Subsystem/Peci to Body ==
  data: Va input; Qa2b input; Vb output
function Vb = EciToBody(Va,Qa2b)
Qb2a = QInv(Qa2b);
qout = QMul(QMul(Qb2a, [0;Va]), Qa2b);
Vb   = [qout(2) qout(3) qout(4)]';

== matlab function fs9_sim_sdr_v0/Sensor Functions/MAG FUNCTION/bdotsdot ==
  data: B input; fsw parameter; bdot output; sdot output
 function [bdot, sdot] =  bdot_sdot(B, fsw)

persistent b_1
B_NORM = norm(B);
b      = B/B_NORM;
if isempty(b_1)
    b_1 = b;
end

bdot = (b-b_1)/fsw.bdot_period;
sdot = (bdot-b*(b'*bdot))/B_NORM;

b_1 = b;

== matlab function fs9_sim_sdr_v0/Spacecraft/Spacecraft Dynamics/Disturbance Models/Subsystem/Veci to Body ==
  data: Va input; Qa2b input; Vb output
function Vb = EciToBody(Va,Qa2b)
Qb2a = QInv(Qa2b);
qout = QMul(QMul(Qb2a, [0;Va]), Qa2b);
Vb   = [qout(2) qout(3) qout(4)]';

== matlab function fs9_sim_sdr_v0/Spacecraft/Spacecraft Dynamics/RigidBody Dynamics/MATLAB Function1 ==
  data: h input; dLdt output size=3; N input; W input; dm parameter
%% Euler Equation
function dLdt = EulerEquation(h,N,W,dm)
L = dm.Ib*W + h;
% dLdt = N-cross((dm.Ib\(L-h)),L);
% L = dm.Ib*W + h;
dLdt = N-cross(W,L);

== matlab function fs9_sim_sdr_v0/Spacecraft/Spacecraft Dynamics/RigidBody Dynamics/MATLAB Function2 ==
  data: h input; W output; L input; dm parameter
%% total angular momentum of the spacecraft
function W = InvTotAngMom(h,L,dm)
W =dm.Ib\(L-h);

== matlab function fs9_sim_sdr_v0/Spacecraft/Spacecraft Dynamics/RigidBody Dynamics/MATLAB Function3 ==
  data: Qi2b input; dQdt output size=4; W input
%% Quaternion Kinematic Equation
function dQdt = QuatKinematic(Qi2b,W)

dQdt = 0.5 * (QMul(Qi2b,[0;W]));

== matlab function fs9_sim_sdr_v0/Space Environment Models/MagneticField/Variant Subsystem/IGRF2020/IGRF_ned2ecef ==
  data: DCM input; Vecef output; Vned input
function Vecef = fcn(DCM,Vned)

Vecef = DCM'*Vned;

== matlab function fs9_sim_sdr_v0/Spacecraft/EPS/DOD Calculation ==
  settings: updateMethod=DISCRETE
  data: eclipse_flag input; dod output; sun_sc input; dm parameter; dod_max output; sa_ang output; batt_io_energy output
function [dod, dod_max,sa_ang, batt_io_energy ] = dod(eclipse_flag, sun_sc, dm)
persistent energy_balance max_dod

%% initializing
max_batt_energy = dm.eps.batt.energy.eol*3600; % J (Joule);
sa_dot = 0;
if isempty(energy_balance)
    energy_balance = 0; 
    max_dod = 0;
end

if isempty(max_dod)
    max_dod = 0;
end

energy_balance = energy_balance- dm.eps.power_used.bus.mean *dm.dt;

if ~eclipse_flag 
    sa_dot = dot(dm.eps.sa.normal, sun_sc);
    if sa_dot >0
        energy_balance = energy_balance + dm.eps.sa.power_gen.max * sa_dot * dm.dt;
    end
end

energy_left = max_batt_energy+energy_balance;
dod         = (1-energy_left/max_batt_energy)*100;

if dod < 0
    dod = 0;
end

if dod > max_dod
    max_dod = dod;
end

sa_ang      = acosd(sa_dot);
batt_io_energy = energy_balance;
dod_max     = max_dod;

== matlab function fs9_sim_sdr_v0/Spacecraft/Spacecraft Dynamics/Disturbance Models/Subsystem/Charge Condition ==
  data: Eclipse input; SunBody input; AngSunNZ output
 function AngSunNZ  = ChargeStatus(Eclipse, SunBody)
NZBody = [0 0 -1];
ang = acosd(dot(SunBody, NZBody));

if ( Eclipse ~= 1 && ang < 90 && ang > 0)
    AngSunNZ = ang;
else
    AngSunNZ = 0;
end

end

== matlab function fs9_sim_sdr_v0/Space Environment Models/Orbit Propagator /J2 Ben ==
  data: X input; Xdot output; dm parameter
function Xdot = J2(X, dm)

r = X(1:3);
v = X(4:6);
J2 = 0.484165143790815D-03*(5)^0.5;
GMe = 3.986004418e14;                % m^3*s^-2
Re = 6378137;                        % earth radius, m
k_1_2 = -GMe/norm(r)^3 * (1+ 1.5 *J2* (Re/norm(r))^2 * (1 - 5* (r(3)/norm(r))^2) );
k_3 = -GMe/norm(r)^3 * (1+ 1.5 *J2* (Re/norm(r))^2 * (3 - 5* (r(3)/norm(r))^2) );
a = [k_1_2*r(1); k_1_2*r(2); k_3*r(3)];
Xdot=[v; a];

% Re   = 6378137.00;%m
% mu_e = 3.986004418e14;%3.986004418e14;
% 
% p = X(1:3);
% v = X(4:6);
% R = norm(p);
% 
% 
% J2 = 0.001082626173852;%0.001082626173852;% C20_bar = -0.484165143790815D-03 from EGM2008
% %0.001082626683553151; STK
%      
% ReOverR_2 = (Re/R)^2;
% sinphi_2   = (p(3)/R)^2;
% muOverR_3 = mu_e/R^3;
% vdot=[-muOverR_3*(1+1.5*J2*ReOverR_2*(1-5*sinphi_2));...
%       -muOverR_3*(1+1.5*J2*ReOverR_2*(1-5*sinphi_2));...
%       -muOverR_3*(1+1.5*J2*ReOverR_2*(3-5*sinphi_2))].*p;
%      
% Xdot=[v; vdot];

== matlab function fs9_sim_sdr_v0/Space Environment Models/Orbit Propagator /J2 Jack ==
  data: X input; Xdot output; dm parameter
function Xdot = J2(X, dm)

Re   = 6378137.00;%m
mu_e = 3.986004418e14;%3.986004418e14;

p = X(1:3);
v = X(4:6);
R = norm(p);


J2 = 0.001082626173852;%0.001082626173852;% C20_bar = -0.484165143790815D-03 from EGM2008
%0.001082626683553151; STK
     
ReOverR_2 = (Re/R)^2;
sinphi_2   = (p(3)/R)^2;
muOverR_3 = mu_e/R^3;
vdot=[-muOverR_3*(1+1.5*J2*ReOverR_2*(1-5*sinphi_2));...
      -muOverR_3*(1+1.5*J2*ReOverR_2*(1-5*sinphi_2));...
      -muOverR_3*(1+1.5*J2*ReOverR_2*(3-5*sinphi_2))].*p;
     
Xdot=[v; vdot];

== matlab function fs9_sim_sdr_v0/RWA/Nonlinear/RW1/MATLAB Function ==
  data: torque input; torque output; rate input; dm parameter
function torque = torqueBox(torque,rate, dm)

momentum = dm.rw_mdl.moi * rate;
maxAngMom = dm.rw_mdl.maxAngMom;
AvlAngMom = dm.rw_mdl.avlAngMom;
maxTorque = dm.rw_mdl.maxTorque;

if momentum >= AvlAngMom && momentum <= maxAngMom
    torque = 1 + (-maxTorque) * (momentum);
elseif momentum <= -AvlAngMom && momentum >= (-maxAngMom)
    torque = -1 + (-maxTorque) * (momentum);
end

== matlab function fs9_sim_sdr_v0/RWA/Nonlinear/RW2/MATLAB Function ==
  data: torque input; torque output; rate input; dm parameter
function torque = torqueBox(torque,rate, dm)

momentum = dm.rw_mdl.moi * rate;
maxAngMom = dm.rw_mdl.maxAngMom;
AvlAngMom = dm.rw_mdl.avlAngMom;
maxTorque = dm.rw_mdl.maxTorque;

if momentum >= AvlAngMom && momentum <= maxAngMom
    torque = 1 + (-maxTorque) * (momentum);
elseif momentum <= -AvlAngMom && momentum >= (-maxAngMom)
    torque = -1 + (-maxTorque) * (momentum);
end

== matlab function fs9_sim_sdr_v0/Space Environment Models/Orbit Propagator /gravityField/TwoBodyRHS/MATLAB Function ==
  data: X input; Xdot output; dm parameter
function Xdot = TwoBodyRHS(X, dm)

r = X(1:3);
v = X(4:6);
Xdot=[v; -(dm.mu_e*r/norm(r)^3)];

== matlab function fs9_sim_sdr_v0/Space Environment Models/Orbit Propagator /gravityField/J2/J2 Jack ==
  data: X input; Xdot output; dm parameter
function Xdot = J2(X, dm)

Re   = 6378137.00;%m
mu_e = 3.986004418e14;%3.986004418e14;

p = X(1:3);
v = X(4:6);
R = norm(p);


J2 = 0.001082626173852;%0.001082626173852;% C20_bar = -0.484165143790815D-03 from EGM2008
%0.001082626683553151; STK
     
ReOverR_2 = (Re/R)^2;
sinphi_2   = (p(3)/R)^2;
muOverR_3 = mu_e/R^3;
vdot=[-muOverR_3*(1+1.5*J2*ReOverR_2*(1-5*sinphi_2));...
      -muOverR_3*(1+1.5*J2*ReOverR_2*(1-5*sinphi_2));...
      -muOverR_3*(1+1.5*J2*ReOverR_2*(3-5*sinphi_2))].*p;
     
Xdot=[v; vdot];

== matlab function fs9_sim_sdr_v0/RWA/Nonlinear/RW3/MATLAB Function ==
  data: torque input; torque output; rate input; dm parameter
function torque = torqueBox(torque,rate, dm)

momentum = dm.rw_mdl.moi * rate;
maxAngMom = dm.rw_mdl.maxAngMom;
AvlAngMom = dm.rw_mdl.avlAngMom;
maxTorque = dm.rw_mdl.maxTorque;

if momentum >= AvlAngMom && momentum <= maxAngMom
    torque = 1 + (-maxTorque) * (momentum);
elseif momentum <= -AvlAngMom && momentum >= (-maxAngMom)
    torque = -1 + (-maxTorque) * (momentum);
end

== matlab function fs9_sim_sdr_v0/RWA/Nonlinear/RW4/MATLAB Function ==
  data: torque input; torque output; rate input; dm parameter
function torque = torqueBox(torque,rate, dm)

momentum = dm.rw_mdl.moi * rate;
maxAngMom = dm.rw_mdl.maxAngMom;
AvlAngMom = dm.rw_mdl.avlAngMom;
maxTorque = dm.rw_mdl.maxTorque;

if momentum >= AvlAngMom && momentum <= maxAngMom
    torque = 1 + (-maxTorque) * (momentum);
elseif momentum <= -AvlAngMom && momentum >= (-maxAngMom)
    torque = -1 + (-maxTorque) * (momentum);
end
